simulink model "controller"  (R2015a)
settings: Solver=ode45  StartTime=0.0  StopTime=10.0  RelTol=1e-3
values from neighbouring files (symbols this model uses):
  params = catstruct(params, sys.params_str)    [double_lqg.m]    (also in load_mechanism_params.m = params(1:13); load_params.m = [g, m0, b0,                m1, I1, b1, L1, L1_cg,           ; load_single_mechanism_params.m = params(1:8); load_single_params.m = [g, m0, b0,                m1, I1, b1, L1, L1_cg,           )
settings Model: Creator=BPeixoto  LastModifiedBy=BPeixoto

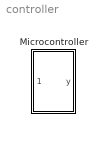
== system controller ==
  Microcontroller : Subsystem

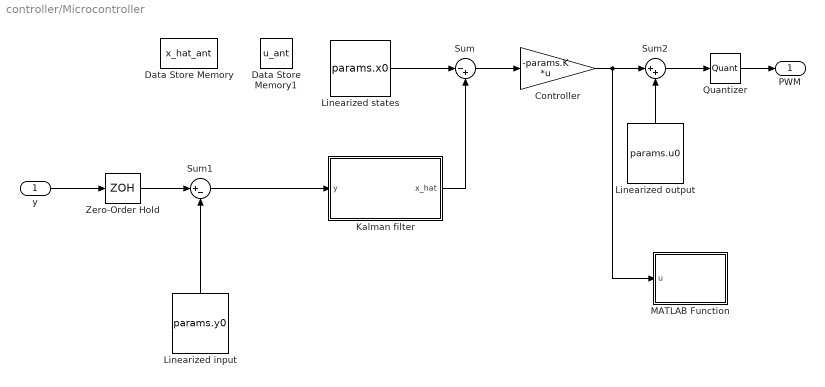
== system controller/Microcontroller ==
  y : Inport
  Controller : Gain  Gain=-params.K  Multiplication=Matrix(K*u)
  Data Store Memory : DataStoreMemory  DataStoreName=x_hat_ant  ReadBeforeWriteMsg=warning  WriteAfterWriteMsg=warning  WriteAfterReadMsg=warning  InitialValue=zeros(6, 1)  OutDataTypeStr=double
  Data Store Memory1 : DataStoreMemory  DataStoreName=u_ant  ReadBeforeWriteMsg=warning  WriteAfterWriteMsg=warning  WriteAfterReadMsg=warning  OutDataTypeStr=double
  Kalman filter : MATLAB Function  TreatAsAtomicUnit=on
  Linearized input : Constant  Value=params.y0
  Linearized output : Constant  Value=params.u0
  Linearized states : Constant  Value=params.x0
  MATLAB Function : MATLAB Function  TreatAsAtomicUnit=on
  Quantizer : Quantizer  QuantizationInterval=1/2^(params.nbits)
  Sum : Sum  Inputs=|-+
  Sum1 : Sum  Inputs=|+-
  Sum2 : Sum  Inputs=|++
  Zero-Order Hold : ZeroOrderHold  SampleTime=params.ts
  PWM : Outport
  wires:
  y/1 -> Zero-Order Hold/1
  Linearized states/1 -> Sum/1
  Sum/1 -> Controller/1
  Linearized input/1 -> Sum1/2
  Zero-Order Hold/1 -> Sum1/1
  Quantizer/1 -> PWM/1
  Controller/1 -> MATLAB Function/1(u), Sum2/1
  Linearized output/1 -> Sum2/2
  Sum2/1 -> Quantizer/1
  Sum1/1 -> Kalman filter/1(y)
  Kalman filter/1(x_hat) -> Sum/2

== matlab function controller/Microcontroller/Kalman filter ==
  data: y input; params parameter; x_hat output; x_hat_ant data_store_memory
function x_hat = kalman_filter(y, params)
    % First assignemnt
    global u_ant;
    global x_hat_ant;
    
    [n, m] = size(params.Gamma);
            
    % Main matrices
    L = params.L;
    Phi = params.Phi;
    Gamma = params.Gamma;
    C = params.C;
    
    % Time and measurement update 
    x_bar = Phi*x_hat_ant + Gamma*u_ant;
    x_hat = x_bar + L*(y - C*x_bar);
    
    % Time update
    x_hat_ant = x_hat;
end

== matlab function controller/Microcontroller/MATLAB Function ==
  data: u input; u_ant data_store_memory
function save_uant(u)    
    global u_ant;    
    u_ant = u;
end
